simulink model "position_estimator_ss"  (R2021a)
settings: Solver=VariableStepDiscrete  StartTime=0.0  StopTime=10.0  RelTol=1e-3
values from neighbouring files (symbols this model uses):
  Ad = [[1, Ts,  -Ts^2*a33] ... (first row only)    [dev_position_estimator.m]    (also in eval_logs.m)
  Bd = [Ts^2 ... (first row only)    [dev_position_estimator.m]    (also in eval_logs.m)
  K = [k1; k2; k3]    [dev_position_estimator.m]    (also in eval_log_40804.m = [k1, k2, k3].'; eval_logs.m)
  nd_pos = 12    [dev_position_estimator.m]    (also in eval_logs.m = 4; test_position_estimator.m = 9)
  Ts = 1/40    (= 0.025)    [check_median.m]    (also in check_pade.m; check_pt3_init.m; dev_position_estimator.m = 0.00833333333333; eval_filter_poles.m = 0.01)
settings Model: Creator=pmic  LastModifiedBy=pmic

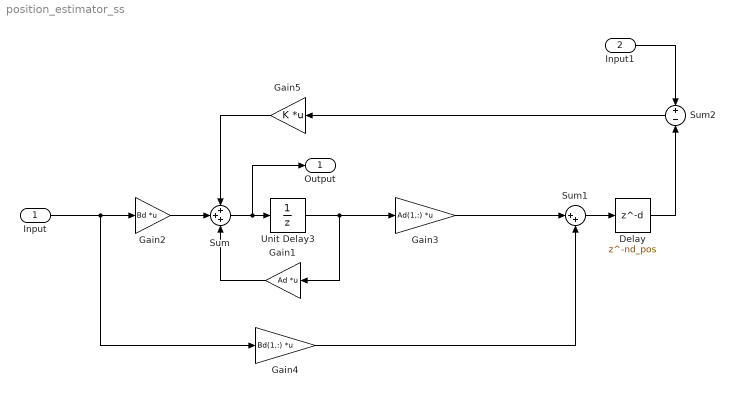
== system position_estimator_ss ==
  Input : Inport
  Input1 : Inport  Port=2
  Delay : Delay  DelayLength=nd_pos  SampleTime=Ts
  Gain1 : Gain  Gain=Ad  Multiplication=Matrix(K*u)
  Gain2 : Gain  Gain=Bd  Multiplication=Matrix(K*u)
  Gain3 : Gain  Gain=Ad(1,:)  Multiplication=Matrix(K*u)
  Gain4 : Gain  Gain=Bd(1,:)  Multiplication=Matrix(K*u)
  Gain5 : Gain  Gain=K  Multiplication=Matrix(K*u)
  Sum : Sum  Inputs=+++
  Sum1 : Sum  Inputs=|++
  Sum2 : Sum  Inputs=+|-
  Unit Delay3 : UnitDelay  SampleTime=Ts  HasFrameUpgradeWarning=on
  Output : Outport
  wires:
  Gain1/1 -> Sum/3
  Sum/1 -> Output/1, Unit Delay3/1
  Unit Delay3/1 -> Gain3/1, Gain1/1
  Input/1 -> Gain4/1, Gain2/1
  Gain4/1 -> Sum1/2
  Sum2/1 -> Gain5/1
  Gain2/1 -> Sum/2
  Gain5/1 -> Sum/1
  Input1/1 -> Sum2/1
  Sum1/1 -> Delay/1
  Gain3/1 -> Sum1/1
  Delay/1 -> Sum2/2
